simulink model "cascadecontrol1"  (Simulink 6.1)
settings: Solver=ode45  StartTime=0.0  StopTime=500  RelTol=1e-3
libraries: simulink_extras x3
settings Model: LastModifiedBy=Administrator
settings DebuggingCC: SolverPrmCheckMsg=warning

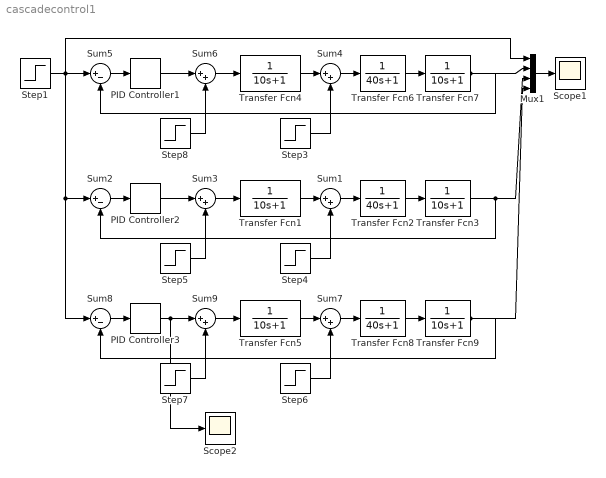
== system cascadecontrol1 ==
  Mux1 : Mux
  PID Controller1 : simulink_extras/Additional Linear/PID Controller  P=4  I=0.05  D=30
  PID Controller2 : simulink_extras/Additional Linear/PID Controller  P=4  I=0.05  D=20
  PID Controller3 : simulink_extras/Additional Linear/PID Controller  P=4  I=0.05  D=30
  Scope1 : Scope
  Scope2 : Scope
  Step1 : Step  Time=0  SampleTime=0
  Step{3..8} (6 alike) : Step  Time=0  After=0  SampleTime=0
  Sum{1,3..4,6..7,9} (6 alike) : Sum  Inputs=|++
  Sum2 : Sum  Inputs=|+-
  Sum5 : Sum  Inputs=|+-
  Sum8 : Sum  Inputs=|+-
  Transfer Fcn{1,3..5,7,9} (6 alike) : TransferFcn  Denominator=[10 1]
  Transfer Fcn2 : TransferFcn  Denominator=[40 1]
  Transfer Fcn6 : TransferFcn  Denominator=[40 1]
  Transfer Fcn8 : TransferFcn  Denominator=[40 1]
  wires:
  Step1/1 -> Mux1/1, Sum5/1, Sum2/1, Sum8/1
  Sum5/1 -> PID Controller1/1
  PID Controller1/1 -> Sum6/1
  Sum4/1 -> Transfer Fcn6/1
  Transfer Fcn7/1 -> Sum5/2, Mux1/2
  Mux1/1 -> Scope1/1
  Sum6/1 -> Transfer Fcn4/1
  Transfer Fcn6/1 -> Transfer Fcn7/1
  Step3/1 -> Sum4/2
  Step8/1 -> Sum6/2
  Transfer Fcn4/1 -> Sum4/1
  Sum2/1 -> PID Controller2/1
  PID Controller2/1 -> Sum3/1
  Sum1/1 -> Transfer Fcn2/1
  Transfer Fcn3/1 -> Sum2/2, Mux1/3
  Sum3/1 -> Transfer Fcn1/1
  Transfer Fcn2/1 -> Transfer Fcn3/1
  Step4/1 -> Sum1/2
  Step5/1 -> Sum3/2
  Transfer Fcn1/1 -> Sum1/1
  Sum8/1 -> PID Controller3/1
  PID Controller3/1 -> Sum9/1, Scope2/1
  Sum7/1 -> Transfer Fcn8/1
  Transfer Fcn9/1 -> Sum8/2, Mux1/4
  Sum9/1 -> Transfer Fcn5/1
  Transfer Fcn8/1 -> Transfer Fcn9/1
  Step6/1 -> Sum7/2
  Step7/1 -> Sum9/2
  Transfer Fcn5/1 -> Sum7/1
